simulink model "hw3_sim_model"  (Simulink 8.0)
settings: Solver=ode23t  StartTime=0.0  StopTime=t_sim  RelTol=1e-3
values from neighbouring files (symbols this model uses):
  alpha1hat = 7    [hw3_problem2.m]
  alpha2hat = 3    [hw3_problem2.m]
  dotxd = 0    [hw3_problem2.m]
  eta = 1    [hw3_problem2.m]
  lambda = 2 * pi    (= 6.28318530718)    [hw3_problem2.m]
  xd = 1    [hw3_problem2.m]
settings Model: Creator=Dan  LastModifiedBy=dpwiese
settings SolverCC: MaxConsecutiveZCs=100  ZeroCrossAlgorithm=Adaptive
settings DataIOCC: SignalLoggingSaveFormat=ModelDataLogs
settings DebuggingCC: FcnCallInpInsideContextMsg=EnableAllAsWarning
settings GRTTargetCC: CombineOutputUpdateFcns=off  GRTInterface=on

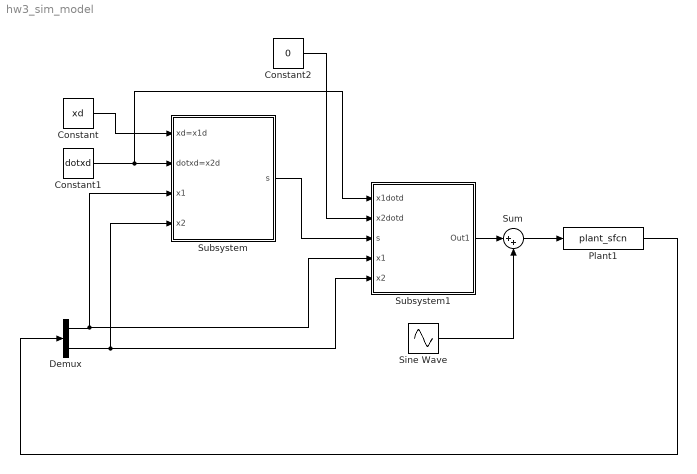
== system hw3_sim_model ==
  Constant : Constant  Value=xd
  Constant1 : Constant  Value=dotxd
  Constant2 : Constant  Value=0
  Demux : Demux  Outputs=2
  Plant1 : S-Function  FunctionName=plant_sfcn  Parameters=startpt  EnableBusSupport=off
  Sine Wave : Sin  Frequency=10  SampleTime=0
  Subsystem : Subsystem
  Subsystem1 : Subsystem
  Sum : Sum  Inputs=|++
  wires:
  Plant1/1 -> Demux/1
  Constant/1 -> Subsystem/1(xd=x1d)
  Constant1/1 -> Subsystem1/1(x1dotd), Subsystem/2(dotxd=x2d)
  Demux/1 -> Subsystem1/4(x1), Subsystem/3(x1)
  Demux/2 -> Subsystem1/5(x2), Subsystem/4(x2)
  Subsystem/1(s) -> Subsystem1/3(s)
  Subsystem1/1(Out1) -> Sum/1
  Sine Wave/1 -> Sum/2
  Sum/1 -> Plant1/1
  Constant2/1 -> Subsystem1/2(x2dotd)

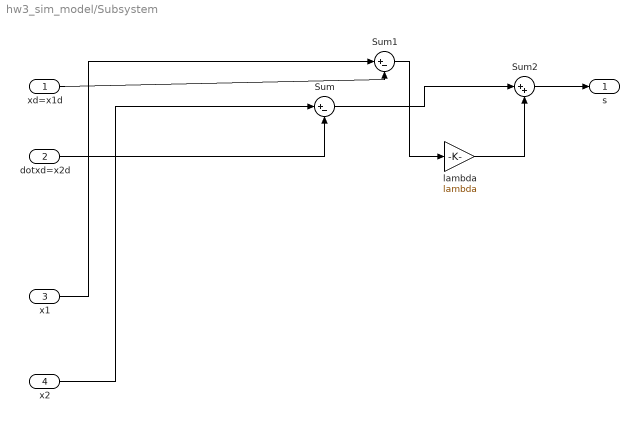
== system hw3_sim_model/Subsystem ==
  xd=x1d : Inport
  dotxd=x2d : Inport  Port=2
  x1 : Inport  Port=3
  x2 : Inport  Port=4
  Sum : Sum  Inputs=|+-
  Sum1 : Sum  Inputs=|+-
  Sum2 : Sum  Inputs=|++
  lambda : Gain  Gain=lambda
  s : Outport
  wires:
  x2/1 -> Sum/1
  dotxd=x2d/1 -> Sum/2
  x1/1 -> Sum1/1
  xd=x1d/1 -> Sum1/2
  Sum/1 -> Sum2/1
  Sum1/1 -> lambda/1
  lambda/1 -> Sum2/2
  Sum2/1 -> s/1

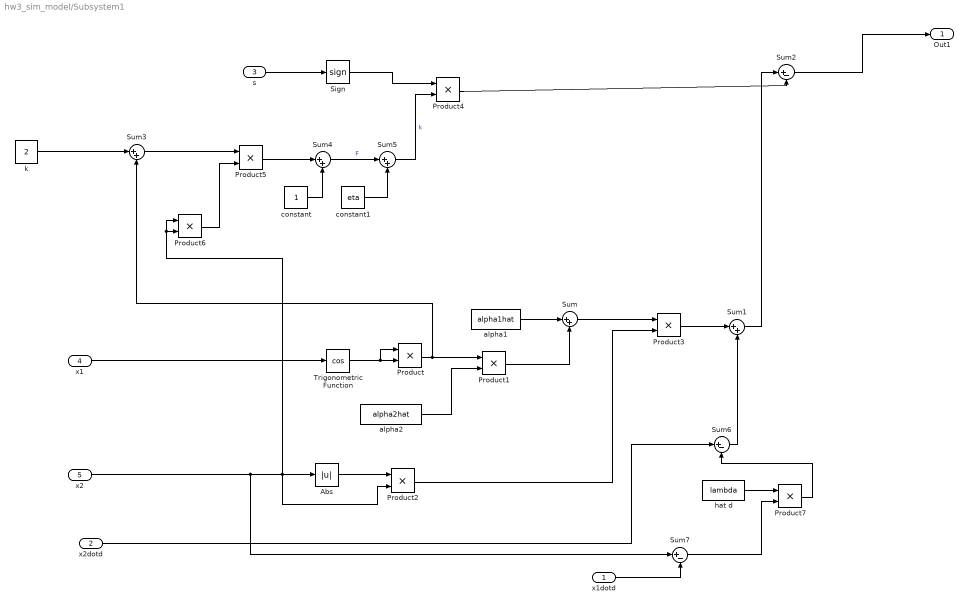
== system hw3_sim_model/Subsystem1 ==
  x1dotd : Inport
  x2dotd : Inport  Port=2
  s : Inport  Port=3
  x1 : Inport  Port=4
  x2 : Inport  Port=5
  Abs : Abs
  Product{,1..7} (8 alike) : Product  RndMeth=Zero
  Sign : Signum
  Sum{,1,3..5} (5 alike) : Sum  Inputs=|++
  Sum2 : Sum  Inputs=|+-
  Sum6 : Sum  Inputs=|+-
  Sum7 : Sum  Inputs=|+-
  Trigonometric Function : Trigonometry  Operator=cos
  alpha1 : Constant  Value=alpha1hat
  alpha2 : Constant  Value=alpha2hat
  constant : Constant
  constant1 : Constant  Value=eta
  hat d : Constant  Value=lambda
  k : Constant  Value=2
  Out1 : Outport
  wires:
  x1/1 -> Trigonometric Function/1
  Trigonometric Function/1 -> Product/2, Product/1
  Product/1 -> Product1/1, Sum3/2
  alpha2/1 -> Product1/2
  alpha1/1 -> Sum/1
  Product1/1 -> Sum/2
  x2/1 -> Sum7/1, Product6/2, Product6/1, Product2/2, Abs/1
  Abs/1 -> Product2/1
  Sum/1 -> Product3/1
  Product2/1 -> Product3/2
  Product3/1 -> Sum1/1
  Sum1/1 -> Sum2/1
  s/1 -> Sign/1
  Sign/1 -> Product4/1
  Product4/1 -> Sum2/2
  Sum2/1 -> Out1/1
  k/1 -> Sum3/1
  Sum3/1 -> Product5/1
  Product6/1 -> Product5/2
  Product5/1 -> Sum4/1
  constant/1 -> Sum4/2
  Sum4/1 -> Sum5/1  "F"
  constant1/1 -> Sum5/2
  Sum5/1 -> Product4/2  "k"
  x2dotd/1 -> Sum6/1
  hat d/1 -> Product7/1
  x1dotd/1 -> Sum7/2
  Sum7/1 -> Product7/2
  Product7/1 -> Sum6/2
  Sum6/1 -> Sum1/2
